simulink model "EngineOnly"  (R2016a)
settings: Solver=VariableStepAuto  StartTime=0.0  StopTime=300.0  RelTol=1e-3
libraries: simulink x1
settings Model: Creator=sid_1  LastModifiedBy=sid_1

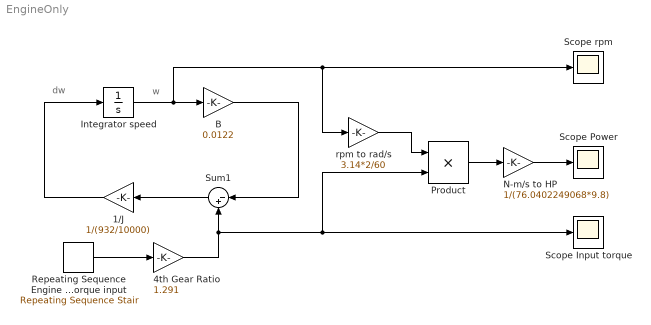
== system EngineOnly ==
  note: w
  note: dw
  1/J : Gain  Gain=1/(932/10000)
  4th Gear Ratio : Gain  Gain=1.291
  B : Gain  Gain=0.0122
  Integrator speed : Integrator
  N-m/s to HP : Gain  Gain=1/(76.0402249068*9.8)
  Product : Product
  Repeating Sequence Engine Torque input : simulink/Sources/Repeating Sequence Stair  OutValues=[1:.45:77 77 77 77 77 77 77 77 77 77 77 77 77 77 77 77 77 77 77 77 77 77 77 77 77 77 77 77 77 77 77 77 77 77 77 77 77 77 77 77 77 77 77 77 77 77 77 77 77 77 77 77 77 77 77 77 77 77 77 77 77 77 77 77 77 77 77 77 77 77 77 77 77 77 77 77 77 77 77 77 77 77 77 77 77 77 77 77 77 77 77 77 77 77 77 77 77 77 77 77 77 77 77 77 77 77 77 77 77 77 77 77 77 77 77 77 77 77 77 77 77 77 77 77 77 77 77 77 77 77 77 77 77 77 77 77 77 77 77 77 77 77 77 77 77 77 77 77 77 77 77 77 77 77 77 77 77 77 77 77 77 77 77 77 77 77 77 77 77 77 77 77 77 77 77 77 77 77]  tsamp=1  OutMin=[]  OutMax=[]  OutDataTypeStr=single  OutputDataTypeScalingMode=single  OutDataType=fixdt(0,8)  ConRadixGroup=Best Precision: Vector-wise  OutScaling=2^-12
  Scope Power : Scope
  Scope rpm : Scope
  Scope Input torque : Scope
  Sum1 : Sum  Inputs=|-+
  rpm to rad/s : Gain  Gain=3.14*2/60
  wires:
  Integrator speed/1 -> rpm to rad/s/1, Scope rpm/1, B/1
  Sum1/1 -> 1/J/1
  Repeating Sequence Engine Torque input/1 -> 4th Gear Ratio/1
  1/J/1 -> Integrator speed/1
  B/1 -> Sum1/1
  4th Gear Ratio/1 -> Sum1/2, Product/2, Scope Input torque/1
  Product/1 -> N-m/s to HP/1
  rpm to rad/s/1 -> Product/1
  N-m/s to HP/1 -> Scope Power/1
